simulink model "Main_C0_C3"  (R2023a)
(part 2 of 37)

  Left T Spine : sm_lib/Body Elements/File Solid  ExtGeomFileName=C:\Users\siril\OneDrive\Desktop\TIM-Control\Matlab\Simscape models\CAD - with COM\SymmetricModel\draft7\LeftThoracicSpineWithRibcage.step  UnitType=FromFile  ExtGeomFileUnits=m  StepReaderType=HEX  ExportConvexHullGeometry=off  InertiaType=CalculateFromGeometry  Mass=1  MassUnits=kg  CenterOfMass=[0 0 0]  CenterOfMassUnits=m  MomentsOfInertia=[1 1 1]  MomentsOfInertiaUnits=kg*m^2  ProductsOfInertia=[0 0 0]  ProductsOfInertiaUnits=kg*m^2  BasedOnType=Density  Density=0.182  DensityUnits=g/cm^3  DoExposeReferenceFrame=off  SerializedFrames=<Frames><Frame><Id>Frame1</Id><Value><Name>To L1</Name><Origin><Source>GeometricFeature</Source><FeatureName>segment 762</FeatureName></Origin><PrimaryAxis><DefinedDirection>-Z</DefinedDirection><Source>GeometricFeature</Source><SourceDirection>+Z</SourceDirection><FeatureName>planar surface 1266</FeatureName></PrimaryAxis><SecondaryAxis><DefinedDirection>+X</DefinedDirection><Source>ReferenceFrame</Source><SourceDirection>+X</SourceDirection><FeatureName></FeatureName></SecondaryAxis></Value></Frame><Frame><Id>Frame2</Id><Value><Name>To Left Abdominal Muscle</Name><Origin><Source>GeometricFeature</Source><FeatureName>planar surface 54556</FeatureName></Origin><PrimaryAxis><DefinedDirection>+Z</DefinedDirection><Source>GeometricFeature</Source><SourceDirection>+Z</SourceDirection><FeatureName>planar surface 54556</FeatureName></PrimaryAxis><SecondaryAxis><DefinedDirection>+X</DefinedDirection><Source>ReferenceFrame</Source><SourceDirection>+X</SourceDirection><FeatureName></FeatureName></SecondaryAxis></Value></Frame><Frame><Id>Frame3</Id><Value><Name>To Left Back Muscle</Name><Origin><Source>GeometricFeature</Source><FeatureName>planar surface 54574</FeatureName></Origin><PrimaryAxis><DefinedDirection>-Z</DefinedDirection><Source>GeometricFeature</Source><SourceDirection>+Z</SourceDirection><FeatureName>planar surface 54574</FeatureName></PrimaryAxis><SecondaryAxis><DefinedDirection>+X</DefinedDirection><Source>ReferenceFrame</Source><SourceDirection>+X</SourceDirection><FeatureName></FeatureName></SecondaryAxis></Value></Frame><Frame><Id>Frame4</Id><Value><Name>To Left Transverse1 Muscle</Name><Origin><Source>GeometricFeature</Source><FeatureName>planar surface 54586</FeatureName></Origin><PrimaryAxis><DefinedDirection>+Z</DefinedDirection><Source>GeometricFeature</Source><SourceDirection>+Z</SourceDirection><FeatureName>planar surface 54586</FeatureName></PrimaryAxis><SecondaryAxis><DefinedDirection>+X</DefinedDirection><Source>ReferenceFrame</Source><SourceDirection>+X</SourceDirection><FeatureName></FeatureName></SecondaryAxis></Value></Frame><Frame><Id>Frame5</Id><Value><Name>To Left Transverse2 Muscle</Name><Origin><Source>GeometricFeature</Source><FeatureName>planar surface 54611</FeatureName></Origin><PrimaryAxis><DefinedDirection>+Z</DefinedDirection><Source>GeometricFeature</Source><SourceDirection>+Z</SourceDirection><FeatureName>planar surface 54611</FeatureName></PrimaryAxis><SecondaryAxis><DefinedDirection>+X</DefinedDirection><Source>ReferenceFrame</Source><SourceDirection>+X</SourceDirection><FeatureName></FeatureName></SecondaryAxis></Value></Frame><Frame><Id>Frame6</Id><Value><Name>E01_Left_End_onTSpine</Name><Origin><Source>GeometricFeature</Source><FeatureName>point 64319</FeatureName></Origin><PrimaryAxis><DefinedDirection>+Z</DefinedDirection><Source>ReferenceFrame</Source><SourceDirection>+Z</SourceDirection><FeatureName></FeatureName></PrimaryAxis><SecondaryAxis><DefinedDirection>+X</DefinedDirection><Source>ReferenceFrame</Source><SourceDirection>+X</SourceDirection><FeatureName></FeatureName></SecondaryAxis></Value></Frame><Frame><Id>Frame7</Id><Value><Name>E02_Left_End_onTSpine</Name><Origin><Source>GeometricFeature</Source><FeatureName>point 57959</FeatureName></Origin><PrimaryAxis><DefinedDirection>+Z</DefinedDirection><Source>ReferenceFrame</Source><SourceDirection>+Z</SourceDirection><FeatureName></FeatureName></PrimaryAxis><SecondaryAxis><DefinedDirection>+X</DefinedDirection><Source>ReferenceFrame</Source><SourceDirection>+X</SourceDirection><FeatureName></FeatureName></SecondaryAxis></Value></Frame><Frame><Id>Frame8</Id><Value><Name>IO1_Left_End_onTSpine</Name><Origin><Source>GeometricFeature</Source><FeatureName>point 6575</FeatureName></Origin><PrimaryAxis><DefinedDirection>+Z</DefinedDirection><Source>ReferenceFrame</Source><SourceDirection>+Z</SourceDirection><FeatureName></FeatureName></PrimaryAxis><SecondaryAxis><DefinedDirection>+X</DefinedDirection><Source>ReferenceFrame</Source><SourceDirection>+X</SourceDirection><FeatureName></FeatureName></SecondaryAxis></Value></Frame><Frame><Id>Frame9</Id><Value><Name>IO2_Left_End_onTSpine</Name><Origin><Source>GeometricFeature</Source><FeatureName>point 61983</FeatureName></Origin><PrimaryAxis><DefinedDirection>+Z</DefinedDirection><Source>ReferenceFrame</Source><SourceDirection>+Z</SourceDirection><FeatureName></FeatureName></PrimaryAxis><SecondaryAxis><DefinedDirection>+X</DefinedDirection><Source>ReferenceFrame</Source><SourceDirection>+X</SourceDirection><FeatureName></FeatureName></SecondaryAxis></Value></Frame><Frame><Id>Frame10</Id><Value><Name>IO3_Left_End_onTSpine</Name><Origin><Source>GeometricFeature</Source><FeatureName>point 63240</FeatureName></Origin><PrimaryAxis><DefinedDirection>+Z</DefinedDirection><Source>ReferenceFrame</Source><SourceDirection>+Z</SourceDirection><FeatureName></FeatureName></PrimaryAxis><SecondaryAxis><DefinedDirection>+X</DefinedDirection><Source>ReferenceFrame</Source><SourceDirection>+X</SourceDirection><FeatureName></FeatureName></SecondaryAxis></Value></Frame><Frame><Id>Frame11</Id><Value><Name>To Left Clavicle</Name><Origin><Source>GeometricFeature</Source><FeatureName>point 134733</FeatureName></Origin><PrimaryAxis><DefinedDirection>+Z</DefinedDirection><Source>ReferenceFrame</Source><SourceDirection>+Z</SourceDirection><FeatureName></FeatureName></PrimaryAxis><SecondaryAxis><DefinedDirection>+X</DefinedDirection><Source>ReferenceFrame</Source><SourceDirection>+X</SourceDirection><FeatureName></FeatureName></SecondaryAxis></Value></Frame><Frame><Id>Frame12</Id><Value><Name>Left Lat1 Wrap1</Name><Origin><Source>GeometricFeature</Source><FeatureName>point 74792</FeatureName></Origin><PrimaryAxis><DefinedDirection>+Z</DefinedDirection><Source>ReferenceFrame</Source><SourceDirection>+Z</SourceDirection><FeatureName></FeatureName></PrimaryAxis><SecondaryAxis><DefinedDirection>+X</DefinedDirection><Source>ReferenceFrame</Source><SourceDirection>+X</SourceDirection><FeatureName></FeatureName></SecondaryAxis></Value></Frame><Frame><Id>Frame13</Id><Value><Name>Left Lat2 Wrap1</Name><Origin><Source>GeometricFeature</Source><FeatureName>point 104537</FeatureName></Origin><PrimaryAxis><DefinedDirection>+Z</DefinedDirection><Source>ReferenceFrame</Source><SourceDirection>+Z</SourceDirection><FeatureName></FeatureName></PrimaryAxis><SecondaryAxis><DefinedDirection>+X</DefinedDirection><Source>ReferenceFrame</Source><SourceDirection>+X</SourceDirection><FeatureName></FeatureName></SecondaryAxis></Value></Frame><Frame><Id>Frame14</Id><Value><Name>Left Lat1 Wrap2</Name><Origin><Source>GeometricFeature</Source><FeatureName>point 107483</FeatureName></Origin><PrimaryAxis><DefinedDirection>+Z</DefinedDirection><Source>ReferenceFrame</Source><SourceDirection>+Z</SourceDirection><FeatureName></FeatureName></PrimaryAxis><SecondaryAxis><DefinedDirection>+X</DefinedDirection><Source>ReferenceFrame</Source><SourceDirection>+X</SourceDirection><FeatureName></FeatureName></SecondaryAxis></Value></Frame><Frame><Id>Frame15</Id><Value><Name>Left Lat2 Wrap2</Name><Origin><Source>GeometricFeature</Source><FeatureName>point 35207</FeatureName></Origin><PrimaryAxis><DefinedDirection>+Z</DefinedDirection><Source>ReferenceFrame</Source><SourceDirection>+Z</SourceDirection><FeatureName></FeatureName></PrimaryAxis><SecondaryAxis><DefinedDirection>+X</DefinedDirection><Source>ReferenceFrame</Source><SourceDirection>+X</SourceDirection><FeatureName></FeatureName></SecondaryAxis></Value></Frame><Frame><Id>Frame16</Id><Value><Name>Left Lat3 Wrap1</Name><Origin><Source>GeometricFeature</Source><FeatureName>point 22410</FeatureName></Origin><PrimaryAxis><DefinedDirection>+Z</DefinedDirection><Source>ReferenceFrame</Source><SourceDirection>+Z</SourceDirection><FeatureName></FeatureName></PrimaryAxis><SecondaryAxis><DefinedDirection>+X</DefinedDirection><Source>ReferenceFrame</Source><SourceDirection>+X</SourceDirection><FeatureName></FeatureName></SecondaryAxis></Value></Frame></Frames>  GraphicType=FromGeometry  MarkerShape=Sphere  MarkerSize=10  GraphicVisPropType=SimpleVisualProperties  GraphicDiffuseColor=[0.84313726 0.8156863 0.7529412]  GraphicSpecularColor=[0.5 0.5 0.5 1.0]  GraphicAmbientColor=[0.15 0.15 0.15 1.0]  GraphicEmissiveColor=[0.0 0.0 0.0 1.0]  GraphicShininess=75  GraphicOpacity=1.0
  Left and Right Intertransverse Ligaments : Subsystem
  Mechanism Configuration : sm_lib/Utilities/Mechanism Configuration  UniformGravity=Constant  GravityVector=[0 0 -9.80665]  GravityVectorUnits=m/s^2  LinearizationDelta=0.001  JointModeTransitionNonlinearIterations=2
  Multiply21 : Gain  Gain=-1
  Muscle Forces : Subsystem
  PS-Simulink Converter{,1..6,8..39} (39 alike) : nesl_utility/PS-Simulink Converter  PhysicalDomain=network_engine_domain  SubClassName=ps_output  LeftPortType=input  RightPortType=output  PseudoPeriodic=off  Frequencies=[]  VectorFormat=inherit  Unit=inherit  AffineConversion=off
  Pure AR Moment at L1 COM : sm_lib/Forces and Torques/External Force and Torque  ForceResolutionFrame=World  EnableForceX=off  EnableForceY=off  EnableForceZ=off  EnableForce=off  TorqueResolutionFrame=World  EnableTorqueX=off  EnableTorqueY=off  EnableTorqueZ=on  EnableTorque=off
  Pure FE Moment at L1 COM : sm_lib/Forces and Torques/External Force and Torque  ForceResolutionFrame=World  EnableForceX=off  EnableForceY=off  EnableForceZ=off  EnableForce=off  TorqueResolutionFrame=World  EnableTorqueX=on  EnableTorqueY=off  EnableTorqueZ=off  EnableTorque=off
  Pure LB Moment at L1 COM : sm_lib/Forces and Torques/External Force and Torque  ForceResolutionFrame=World  EnableForceX=off  EnableForceY=off  EnableForceZ=off  EnableForce=off  TorqueResolutionFrame=World  EnableTorqueX=off  EnableTorqueY=on  EnableTorqueZ=off  EnableTorque=off
  Radians to Degrees3 : simulink_extras/Transformations/Radians to Degrees
  Radians to Degrees9 : simulink_extras/Transformations/Radians to Degrees
  Right T Spine : sm_lib/Body Elements/File Solid  ExtGeomFileName=C:\Users\siril\OneDrive\Desktop\TIM-Control\Matlab\Simscape models\CAD - with COM\SymmetricModel\draft7\RightThoracicSpineWithRibcage.step  UnitType=FromFile  ExtGeomFileUnits=m  StepReaderType=HEX  ExportConvexHullGeometry=off  InertiaType=CalculateFromGeometry  Mass=1  MassUnits=kg  CenterOfMass=[0 0 0]  CenterOfMassUnits=m  MomentsOfInertia=[1 1 1]  MomentsOfInertiaUnits=kg*m^2  ProductsOfInertia=[0 0 0]  ProductsOfInertiaUnits=kg*m^2  BasedOnType=Density  Density=0.182  DensityUnits=g/cm^3  DoExposeReferenceFrame=off  SerializedFrames=<Frames><Frame><Id>Frame1</Id><Value><Name>To L1</Name><Origin><Source>GeometricFeature</Source><FeatureName>segment 633</FeatureName></Origin><PrimaryAxis><DefinedDirection>+Z</DefinedDirection><Source>GeometricFeature</Source><SourceDirection>+Z</SourceDirection><FeatureName>planar surface 1266</FeatureName></PrimaryAxis><SecondaryAxis><DefinedDirection>+X</DefinedDirection><Source>ReferenceFrame</Source><SourceDirection>+X</SourceDirection><FeatureName></FeatureName></SecondaryAxis></Value></Frame><Frame><Id>Frame2</Id><Value><Name>To Right Abdominal Muscle</Name><Origin><Source>GeometricFeature</Source><FeatureName>planar surface 54556</FeatureName></Origin><PrimaryAxis><DefinedDirection>-Z</DefinedDirection><Source>GeometricFeature</Source><SourceDirection>+Z</SourceDirection><FeatureName>planar surface 54556</FeatureName></PrimaryAxis><SecondaryAxis><DefinedDirection>+X</DefinedDirection><Source>ReferenceFrame</Source><SourceDirection>+X</SourceDirection><FeatureName></FeatureName></SecondaryAxis></Value></Frame><Frame><Id>Frame3</Id><Value><Name>To Right Back Muscle</Name><Origin><Source>GeometricFeature</Source><FeatureName>planar surface 54574</FeatureName></Origin><PrimaryAxis><DefinedDirection>+Z</DefinedDirection><Source>GeometricFeature</Source><SourceDirection>+Z</SourceDirection><FeatureName>planar surface 54574</FeatureName></PrimaryAxis><SecondaryAxis><DefinedDirection>+X</DefinedDirection><Source>ReferenceFrame</Source><SourceDirection>+X</SourceDirection><FeatureName></FeatureName></SecondaryAxis></Value></Frame><Frame><Id>Frame4</Id><Value><Name>To Right Transverse1 Muscle</Name><Origin><Source>GeometricFeature</Source><FeatureName>planar surface 54586</FeatureName></Origin><PrimaryAxis><DefinedDirection>-Z</DefinedDirection><Source>GeometricFeature</Source><SourceDirection>+Z</SourceDirection><FeatureName>planar surface 54586</FeatureName></PrimaryAxis><SecondaryAxis><DefinedDirection>+X</DefinedDirection><Source>ReferenceFrame</Source><SourceDirection>+X</SourceDirection><FeatureName></FeatureName></SecondaryAxis></Value></Frame><Frame><Id>Frame5</Id><Value><Name>To Right Transverse2 Muscle</Name><Origin><Source>GeometricFeature</Source><FeatureName>planar surface 54611</FeatureName></Origin><PrimaryAxis><DefinedDirection>-Z</DefinedDirection><Source>GeometricFeature</Source><SourceDirection>+Z</SourceDirection><FeatureName>planar surface 54611</FeatureName></PrimaryAxis><SecondaryAxis><DefinedDirection>+X</DefinedDirection><Source>ReferenceFrame</Source><SourceDirection>+X</SourceDirection><FeatureName></FeatureName></SecondaryAxis></Value></Frame><Frame><Id>Frame6</Id><Value><Name>T1 Plumbline Frame</Name><Origin><Source>GeometricFeature</Source><FeatureName>point 5793</FeatureName></Origin><PrimaryAxis><DefinedDirection>+Z</DefinedDirection><Source>ReferenceFrame</Source><SourceDirection>+Z</SourceDirection><FeatureName></FeatureName></PrimaryAxis><SecondaryAxis><DefinedDirection>+X</DefinedDirection><Source>ReferenceFrame</Source><SourceDirection>+X</SourceDirection><FeatureName></FeatureName></SecondaryAxis></Value></Frame><Frame><Id>Frame7</Id><Value><Name>T5 Spinous Process Tip</Name><Origin><Source>GeometricFeature</Source><FeatureName>point 6426</FeatureName></Origin><PrimaryAxis><DefinedDirection>+Z</DefinedDirection><Source>ReferenceFrame</Source><SourceDirection>+Z</SourceDirection><FeatureName></FeatureName></PrimaryAxis><SecondaryAxis><DefinedDirection>+X</DefinedDirection><Source>ReferenceFrame</Source><SourceDirection>+X</SourceDirection><FeatureName></FeatureName></SecondaryAxis></Value></Frame><Frame><Id>Frame8</Id><Value><Name>T1 Spinous Process Tip</Name><Origin><Source>GeometricFeature</Source><FeatureName>point 327</FeatureName></Origin><PrimaryAxis><DefinedDirection>+Z</DefinedDirection><Source>ReferenceFrame</Source><SourceDirection>+Z</SourceDirection><FeatureName></FeatureName></PrimaryAxis><SecondaryAxis><DefinedDirection>+X</DefinedDirection><Source>ReferenceFrame</Source><SourceDirection>+X</SourceDirection><FeatureName></FeatureName></SecondaryAxis></Value></Frame><Frame><Id>Frame9</Id><Value><Name>T10 Spinous process tip</Name><Origin><Source>GeometricFeature</Source><FeatureName>point 46212</FeatureName></Origin><PrimaryAxis><DefinedDirection>+Z</DefinedDirection><Source>ReferenceFrame</Source><SourceDirection>+Z</SourceDirection><FeatureName></FeatureName></PrimaryAxis><SecondaryAxis><DefinedDirection>+X</DefinedDirection><Source>ReferenceFrame</Source><SourceDirection>+X</SourceDirection><FeatureName></FeatureName></SecondaryAxis></Value></Frame><Frame><Id>Frame10</Id><Value><Name>T12 Spinous Process tip</Name><Origin><Source>GeometricFeature</Source><FeatureName>point 4338</FeatureName></Origin><PrimaryAxis><DefinedDirection>+Z</DefinedDirection><Source>ReferenceFrame</Source><SourceDirection>+Z</SourceDirection><FeatureName></FeatureName></PrimaryAxis><SecondaryAxis><DefinedDirection>+X</DefinedDirection><Source>ReferenceFrame</Source><SourceDirection>+X</SourceDirection><FeatureName></FeatureName></SecondaryAxis></Value></Frame><Frame><Id>Frame11</Id><Value><Name>E01_Right_End_onTSpine</Name><Origin><Source>GeometricFeature</Source><FeatureName>point 58766</FeatureName></Origin><PrimaryAxis><DefinedDirection>+Z</DefinedDirection><Source>ReferenceFrame</Source><SourceDirection>+Z</SourceDirection><FeatureName></FeatureName></PrimaryAxis><SecondaryAxis><DefinedDirection>+X</DefinedDirection><Source>ReferenceFrame</Source><SourceDirection>+X</SourceDirection><FeatureName></FeatureName></SecondaryAxis></Value></Frame><Frame><Id>Frame12</Id><Value><Name>E02_Right_End_onTSpine</Name><Origin><Source>GeometricFeature</Source><FeatureName>point 57959</FeatureName></Origin><PrimaryAxis><DefinedDirection>+Z</DefinedDirection><Source>ReferenceFrame</Source><SourceDirection>+Z</SourceDirection><FeatureName></FeatureName></PrimaryAxis><SecondaryAxis><DefinedDirection>+X</DefinedDirection><Source>ReferenceFrame</Source><SourceDirection>+X</SourceDirection><FeatureName></FeatureName></SecondaryAxis></Value></Frame><Frame><Id>Frame13</Id><Value><Name>IO1_Right_End_onTSpine</Name><Origin><Source>GeometricFeature</Source><FeatureName>point 6577</FeatureName></Origin><PrimaryAxis><DefinedDirection>+Z</DefinedDirection><Source>ReferenceFrame</Source><SourceDirection>+Z</SourceDirection><FeatureName></FeatureName></PrimaryAxis><SecondaryAxis><DefinedDirection>+X</DefinedDirection><Source>ReferenceFrame</Source><SourceDirection>+X</SourceDirection><FeatureName></FeatureName></SecondaryAxis></Value></Frame><Frame><Id>Frame14</Id><Value><Name>IO2_Right_End_onTSpine</Name><Origin><Source>GeometricFeature</Source><FeatureName>point 61985</FeatureName></Origin><PrimaryAxis><DefinedDirection>+Z</DefinedDirection><Source>ReferenceFrame</Source><SourceDirection>+Z</SourceDirection><FeatureName></FeatureName></PrimaryAxis><SecondaryAxis><DefinedDirection>+X</DefinedDirection><Source>ReferenceFrame</Source><SourceDirection>+X</SourceDirection><FeatureName></FeatureName></SecondaryAxis></Value></Frame><Frame><Id>Frame15</Id><Value><Name>IO3_Right_End_onTSpine</Name><Origin><Source>GeometricFeature</Source><FeatureName>point 63240</FeatureName></Origin><PrimaryAxis><DefinedDirection>+Z</DefinedDirection><Source>ReferenceFrame</Source><SourceDirection>+Z</SourceDirection><FeatureName></FeatureName></PrimaryAxis><SecondaryAxis><DefinedDirection>+X</DefinedDirection><Source>ReferenceFrame</Source><SourceDirection>+X</SourceDirection><FeatureName></FeatureName></SecondaryAxis></Value></Frame><Frame><Id>Frame16</Id><Value><Name>To Clavicle</Name><Origin><Source>GeometricFeature</Source><FeatureName>point 134734</FeatureName></Origin><PrimaryAxis><DefinedDirection>+Z</DefinedDirection><Source>ReferenceFrame</Source><SourceDirection>+Z</SourceDirection><FeatureName></FeatureName></PrimaryAxis><SecondaryAxis><DefinedDirection>+X</DefinedDirection><Source>ReferenceFrame</Source><SourceDirection>+X</SourceDirection><FeatureName></FeatureName></SecondaryAxis></Value></Frame><Frame><Id>Frame18</Id><Value><Name>Right Lat2 Wrap1</Name><Origin><Source>GeometricFeature</Source><FeatureName>point 104540</FeatureName></Origin><PrimaryAxis><DefinedDirection>+Z</DefinedDirection><Source>ReferenceFrame</Source><SourceDirection>+Z</SourceDirection><FeatureName></FeatureName></PrimaryAxis><SecondaryAxis><DefinedDirection>+X</DefinedDirection><Source>ReferenceFrame</Source><SourceDirection>+X</SourceDirection><FeatureName></FeatureName></SecondaryAxis></Value></Frame><Frame><Id>Frame19</Id><Value><Name>Right Lat3 Wrap1</Name><Origin><Source>GeometricFeature</Source><FeatureName>point 112273</FeatureName></Origin><PrimaryAxis><DefinedDirection>+Z</DefinedDirection><Source>ReferenceFrame</Source><SourceDirection>+Z</SourceDirection><FeatureName></FeatureName></PrimaryAxis><SecondaryAxis><DefinedDirection>+X</DefinedDirection><Source>ReferenceFrame</Source><SourceDirection>+X</SourceDirection><FeatureName></FeatureName></SecondaryAxis></Value></Frame><Frame><Id>Frame20</Id><Value><Name>Right Lat1 Wrap1</Name><Origin><Source>GeometricFeature</Source><FeatureName>point 74799</FeatureName></Origin><PrimaryAxis><DefinedDirection>+Z</DefinedDirection><Source>ReferenceFrame</Source><SourceDirection>+Z</SourceDirection><FeatureName></FeatureName></PrimaryAxis><SecondaryAxis><DefinedDirection>+X</DefinedDirection><Source>ReferenceFrame</Source><SourceDirection>+X</SourceDirection><FeatureName></FeatureName></SecondaryAxis></Value></Frame><Frame><Id>Frame21</Id><Value><Name>Right Lat2 Wrap2</Name><Origin><Source>GeometricFeature</Source><FeatureName>point 35221</FeatureName></Origin><PrimaryAxis><DefinedDirection>+Z</DefinedDirection><Source>ReferenceFrame</Source><SourceDirection>+Z</SourceDirection><FeatureName></FeatureName></PrimaryAxis><SecondaryAxis><DefinedDirection>+X</DefinedDirection><Source>ReferenceFrame</Source><SourceDirection>+X</SourceDirection><FeatureName></FeatureName></SecondaryAxis></Value></Frame><Frame><Id>Frame22</Id><Value><Name>Right Lat1 Wrap2</Name><Origin><Source>GeometricFeature</Source><FeatureName>point 107483</FeatureName></Origin><PrimaryAxis><DefinedDirection>+Z</DefinedDirection><Source>ReferenceFrame</Source><SourceDirection>+Z</SourceDirection><FeatureName></FeatureName></PrimaryAxis><SecondaryAxis><DefinedDirection>+X</DefinedDirection><Source>ReferenceFrame</Source><SourceDirection>+X</SourceDirection><FeatureName></FeatureName></SecondaryAxis></Value></Frame></Frames>  GraphicType=FromGeometry  MarkerShape=Sphere  MarkerSize=10  GraphicVisPropType=SimpleVisualProperties  GraphicDiffuseColor=[0.84313726 0.8156863 0.7529412]  GraphicSpecularColor=[0.5 0.5 0.5 1.0]  GraphicAmbientColor=[0.15 0.15 0.15 1.0]  GraphicEmissiveColor=[0.0 0.0 0.0 1.0]  GraphicShininess=75  GraphicOpacity=1.0
  S1 : sm_lib/Body Elements/File Solid  ExtGeomFileName=C:\Users\siril\OneDrive\Desktop\TIM-Control\Matlab\Simscape models\Reduced Order Model\CAD\model without nucleus\S1.step  UnitType=FromFile  ExtGeomFileUnits=m  StepReaderType=HEX  ExportConvexHullGeometry=off  InertiaType=CalculateFromGeometry  Mass=1  MassUnits=kg  CenterOfMass=[0 0 0]  CenterOfMassUnits=m  MomentsOfInertia=[1 1 1]  MomentsOfInertiaUnits=kg*m^2  ProductsOfInertia=[0 0 0]  ProductsOfInertiaUnits=kg*m^2  BasedOnType=Density  Density=0.182  DensityUnits=g/cm^3  DoExposeReferenceFrame=on  SerializedFrames=<Frames><Frame><Id>Frame1</Id><Value><Name>to IVD5</Name><Origin><Source>GeometricFeature</Source><FeatureName>planar surface 12322</FeatureName></Origin><PrimaryAxis><DefinedDirection>+Z</DefinedDirection><Source>GeometricFeature</Source><SourceDirection>+Z</SourceDirection><FeatureName>planar surface 12322</FeatureName></PrimaryAxis><SecondaryAxis><DefinedDirection>+X</DefinedDirection><Source>ReferenceFrame</Source><SourceDirection>+X</SourceDirection><FeatureName></FeatureName></SecondaryAxis></Value></Frame><Frame><Id>Frame2</Id><Value><Name>For Plumbline Evaluation</Name><Origin><Source>GeometricFeature</Source><FeatureName>planar surface 2453</FeatureName></Origin><PrimaryAxis><DefinedDirection>+Y</DefinedDirection><Source>GeometricFeature</Source><SourceDirection>+Z</SourceDirection><FeatureName>planar surface 2453</FeatureName></PrimaryAxis><SecondaryAxis><DefinedDirection>+X</DefinedDirection><Source>ReferenceFrame</Source><SourceDirection>+X</SourceDirection><FeatureName></FeatureName></SecondaryAxis></Value></Frame><Frame><Id>Frame3</Id><Value><Name>To Right Abdominal Muscle</Name><Origin><Source>GeometricFeature</Source><FeatureName>planar surface 11971</FeatureName></Origin><PrimaryAxis><DefinedDirection>-Z</DefinedDirection><Source>GeometricFeature</Source><SourceDirection>+Z</SourceDirection><FeatureName>planar surface 11971</FeatureName></PrimaryAxis><SecondaryAxis><DefinedDirection>+X</DefinedDirection><Source>ReferenceFrame</Source><SourceDirection>+X</SourceDirection><FeatureName></FeatureName></SecondaryAxis></Value></Frame><Frame><Id>Frame4</Id><Value><Name>To Right Transverse2 Muscle</Name><Origin><Source>GeometricFeature</Source><FeatureName>planar surface 39</FeatureName></Origin><PrimaryAxis><DefinedDirection>-Z</DefinedDirection><Source>GeometricFeature</Source><SourceDirection>+Z</SourceDirection><FeatureName>planar surface 39</FeatureName></PrimaryAxis><SecondaryAxis><DefinedDirection>+X</DefinedDirection><Source>ReferenceFrame</Source><SourceDirection>+X</SourceDirection><FeatureName></FeatureName></SecondaryAxis></Value></Frame><Frame><Id>Frame5</Id><Value><Name>To Right Transverse1 Muscle</Name><Origin><Source>GeometricFeature</Source><FeatureName>planar surface 53</FeatureName></Origin><PrimaryAxis><DefinedDirection>-Z</DefinedDirection><Source>GeometricFeature</Source><SourceDirection>+Z</SourceDirection><FeatureName>planar surface 53</FeatureName></PrimaryAxis><SecondaryAxis><DefinedDirection>+X</DefinedDirection><Source>ReferenceFrame</Source><SourceDirection>+X</SourceDirection><FeatureName></FeatureName></SecondaryAxis></Value></Frame><Frame><Id>Frame6</Id><Value><Name>To Right Back Muscle</Name><Origin><Source>GeometricFeature</Source><FeatureName>planar surface 11999</FeatureName></Origin><PrimaryAxis><DefinedDirection>-Z</DefinedDirection><Source>GeometricFeature</Source><SourceDirection>+Z</SourceDirection><FeatureName>planar surface 11999</FeatureName></PrimaryAxis><SecondaryAxis><DefinedDirection>+X</DefinedDirection><Source>ReferenceFrame</Source><SourceDirection>+X</SourceDirection><FeatureName></FeatureName></SecondaryAxis></Value></Frame><Frame><Id>Frame7</Id><Value><Name>To Left Back Muscle</Name><Origin><Source>GeometricFeature</Source><FeatureName>planar surface 7087</FeatureName></Origin><PrimaryAxis><DefinedDirection>+Z</DefinedDirection><Source>GeometricFeature</Source><SourceDirection>+Z</SourceDirection><FeatureName>planar surface 7087</FeatureName></PrimaryAxis><SecondaryAxis><DefinedDirection>+X</DefinedDirection><Source>ReferenceFrame</Source><SourceDirection>+X</SourceDirection><FeatureName></FeatureName></SecondaryAxis></Value></Frame><Frame><Id>Frame8</Id><Value><Name>To Left Transverse1 Muscle</Name><Origin><Source>GeometricFeature</Source><FeatureName>planar surface 2357</FeatureName></Origin><PrimaryAxis><DefinedDirection>+Z</DefinedDirection><Source>GeometricFeature</Source><SourceDirection>+Z</SourceDirection><FeatureName>planar surface 2357</FeatureName></PrimaryAxis><SecondaryAxis><DefinedDirection>+X</DefinedDirection><Source>ReferenceFrame</Source><SourceDirection>+X</SourceDirection><FeatureName></FeatureName></SecondaryAxis></Value></Frame><Frame><Id>Frame9</Id><Value><Name>To Left Transverse2 Muscle</Name><Origin><Source>GeometricFeature</Source><FeatureName>planar surface 2371</FeatureName></Origin><PrimaryAxis><DefinedDirection>+Z</DefinedDirection><Source>GeometricFeature</Source><SourceDirection>+Z</SourceDirection><FeatureName>planar surface 2371</FeatureName></PrimaryAxis><SecondaryAxis><DefinedDirection>+X</DefinedDirection><Source>ReferenceFrame</Source><SourceDirection>+X</SourceDirection><FeatureName></FeatureName></SecondaryAxis></Value></Frame><Frame><Id>Frame10</Id><Value><Name>To Left Abdominal Muscle</Name><Origin><Source>GeometricFeature</Source><FeatureName>planar surface 7059</FeatureName></Origin><PrimaryAxis><DefinedDirection>+Z</DefinedDirection><Source>GeometricFeature</Source><SourceDirection>+Z</SourceDirection><FeatureName>planar surface 7059</FeatureName></PrimaryAxis><SecondaryAxis><DefinedDirection>+X</DefinedDirection><Source>ReferenceFrame</Source><SourceDirection>+X</SourceDirection><FeatureName></FeatureName></SecondaryAxis></Value></Frame><Frame><Id>Frame11</Id><Value><Name>To L5 SSL</Name><Origin><Source>GeometricFeature</Source><FeatureName>point 40698</FeatureName></Origin><PrimaryAxis><DefinedDirection>+Z</DefinedDirection><Source>ReferenceFrame</Source><SourceDirection>+Z</SourceDirection><FeatureName></FeatureName></PrimaryAxis><SecondaryAxis><DefinedDirection>+X</DefinedDirection><Source>ReferenceFrame</Source><SourceDirection>+X</SourceDirection><FeatureName></FeatureName></SecondaryAxis></Value></Frame><Frame><Id>Frame12</Id><Value><Name>To L5 ISL</Name><Origin><Source>GeometricFeature</Source><FeatureName>point 40776</FeatureName></Origin><PrimaryAxis><DefinedDirection>+Z</DefinedDirection><Source>ReferenceFrame</Source><SourceDirection>+Z</SourceDirection><FeatureName></FeatureName></PrimaryAxis><SecondaryAxis><DefinedDirection>+X</DefinedDirection><Source>ReferenceFrame</Source><SourceDirection>+X</SourceDirection><FeatureName></FeatureName></SecondaryAxis></Value></Frame><Frame><Id>Frame13</Id><Value><Name>To Right L5 ITL</Name><Origin><Source>GeometricFeature</Source><FeatureName>point 2768</FeatureName></Origin><PrimaryAxis><DefinedDirection>+Z</DefinedDirection><Source>ReferenceFrame</Source><SourceDirection>+Z</SourceDirection><FeatureName></FeatureName></PrimaryAxis><SecondaryAxis><DefinedDirection>+X</DefinedDirection><Source>ReferenceFrame</Source><SourceDirection>+X</SourceDirection><FeatureName></FeatureName></SecondaryAxis></Value></Frame><Frame><Id>Frame14</Id><Value><Name>To Left L5 ITL</Name><Origin><Source>GeometricFeature</Source><FeatureName>point 5454</FeatureName></Origin><PrimaryAxis><DefinedDirection>+Z</DefinedDirection><Source>ReferenceFrame</Source><SourceDirection>+Z</SourceDirection><FeatureName></FeatureName></PrimaryAxis><SecondaryAxis><DefinedDirection>+X</DefinedDirection><Source>ReferenceFrame</Source><SourceDirection>+X</SourceDirection><FeatureName></FeatureName></SecondaryAxis></Value></Frame><Frame><Id>Frame15</Id><Value><Name>EO1_Left_Start_onS1</Name><Origin><Source>GeometricFeature</Source><FeatureName>point 6853</FeatureName></Origin><PrimaryAxis><DefinedDirection>+Z</DefinedDirection><Source>ReferenceFrame</Source><SourceDirection>+Z</SourceDirection><FeatureName></FeatureName></PrimaryAxis><SecondaryAxis><DefinedDirection>+X</DefinedDirection><Source>ReferenceFrame</Source><SourceDirection>+X</SourceDirection><FeatureName></FeatureName></SecondaryAxis></Value></Frame><Frame><Id>Frame16</Id><Value><Name>EO2_Left_Start_onS1</Name><Origin><Source>GeometricFeature</Source><FeatureName>point 6794</FeatureName></Origin><PrimaryAxis><DefinedDirection>+Z</DefinedDirection><Source>ReferenceFrame</Source><SourceDirection>+Z</SourceDirection><FeatureName></FeatureName></PrimaryAxis><SecondaryAxis><DefinedDirection>+X</DefinedDirection><Source>ReferenceFrame</Source><SourceDirection>+X</SourceDirection><FeatureName></FeatureName></SecondaryAxis></Value></Frame><Frame><Id>Frame17</Id><Value><Name>EO1_Right_Start_onS1</Name><Origin><Source>GeometricFeature</Source><FeatureName>point 1489</FeatureName></Origin><PrimaryAxis><DefinedDirection>+Z</DefinedDirection><Source>ReferenceFrame</Source><SourceDirection>+Z</SourceDirection><FeatureName></FeatureName></PrimaryAxis><SecondaryAxis><DefinedDirection>+X</DefinedDirection><Source>ReferenceFrame</Source><SourceDirection>+X</SourceDirection><FeatureName></FeatureName></SecondaryAxis></Value></Frame><Frame><Id>Frame18</Id><Value><Name>EO2_Right_Start_onS1</Name><Origin><Source>GeometricFeature</Source><FeatureName>point 1411</FeatureName></Origin><PrimaryAxis><DefinedDirection>+Z</DefinedDirection><Source>ReferenceFrame</Source><SourceDirection>+Z</SourceDirection><FeatureName></FeatureName></PrimaryAxis><SecondaryAxis><DefinedDirection>+X</DefinedDirection><Source>ReferenceFrame</Source><SourceDirection>+X</SourceDirection><FeatureName></FeatureName></SecondaryAxis></Value></Frame><Frame><Id>Frame19</Id><Value><Name>IO1_Right_Start_onS1</Name><Origin><Source>GeometricFeature</Source><FeatureName>point 1008</FeatureName></Origin><PrimaryAxis><DefinedDirection>+Z</DefinedDirection><Source>ReferenceFrame</Source><SourceDirection>+Z</SourceDirection><FeatureName></FeatureName></PrimaryAxis><SecondaryAxis><DefinedDirection>+X</DefinedDirection><Source>ReferenceFrame</Source><SourceDirection>+X</SourceDirection><FeatureName></FeatureName></SecondaryAxis></Value></Frame><Frame><Id>Frame20</Id><Value><Name>IO2_Right_Start_onS1</Name><Origin><Source>GeometricFeature</Source><FeatureName>point 1849</FeatureName></Origin><PrimaryAxis><DefinedDirection>+Z</DefinedDirection><Source>ReferenceFrame</Source><SourceDirection>+Z</SourceDirection><FeatureName></FeatureName></PrimaryAxis><SecondaryAxis><DefinedDirection>+X</DefinedDirection><Source>ReferenceFrame</Source><SourceDirection>+X</SourceDirection><FeatureName></FeatureName></SecondaryAxis></Value></Frame><Frame><Id>Frame21</Id><Value><Name>IO3_Right_Start_onS1</Name><Origin><Source>GeometricFeature</Source><FeatureName>point 1461</FeatureName></Origin><PrimaryAxis><DefinedDirection>+Z</DefinedDirection><Source>ReferenceFrame</Source><SourceDirection>+Z</SourceDirection><FeatureName></FeatureName></PrimaryAxis><SecondaryAxis><DefinedDirection>+X</DefinedDirection><Source>ReferenceFrame</Source><SourceDirection>+X</SourceDirection><FeatureName></FeatureName></SecondaryAxis></Value></Frame><Frame><Id>Frame22</Id><Value><Name>IO1_Left_Start_onS1</Name><Origin><Source>GeometricFeature</Source><FeatureName>point 6435</FeatureName></Origin><PrimaryAxis><DefinedDirection>+Z</DefinedDirection><Source>ReferenceFrame</Source><SourceDirection>+Z</SourceDirection><FeatureName></FeatureName></PrimaryAxis><SecondaryAxis><DefinedDirection>+X</DefinedDirection><Source>ReferenceFrame</Source><SourceDirection>+X</SourceDirection><FeatureName></FeatureName></SecondaryAxis></Value></Frame><Frame><Id>Frame23</Id><Value><Name>IO2_Left_Start_onS1</Name><Origin><Source>GeometricFeature</Source><FeatureName>point 6377</FeatureName></Origin><PrimaryAxis><DefinedDirection>+Z</DefinedDirection><Source>ReferenceFrame</Source><SourceDirection>+Z</SourceDirection><FeatureName></FeatureName></PrimaryAxis><SecondaryAxis><DefinedDirection>+X</DefinedDirection><Source>ReferenceFrame</Source><SourceDirection>+X</SourceDirection><FeatureName></FeatureName></SecondaryAxis></Value></Frame><Frame><Id>Frame24</Id><Value><Name>IO3_Left_Start_onS1</Name><Origin><Source>GeometricFeature</Source><FeatureName>point 6825</FeatureName></Origin><PrimaryAxis><DefinedDirection>+Z</DefinedDirection><Source>ReferenceFrame</Source><SourceDirection>+Z</SourceDirection><FeatureName></FeatureName></PrimaryAxis><SecondaryAxis><DefinedDirection>+X</DefinedDirection><Source>ReferenceFrame</Source><SourceDirection>+X</SourceDirection><FeatureName></FeatureName></SecondaryAxis></Value></Frame></Frames>  GraphicType=FromGeometry  MarkerShape=Sphere  MarkerSize=10  GraphicVisPropType=SimpleVisualProperties  GraphicDiffuseColor=[0.84313726 0.8156863 0.7529412]  GraphicSpecularColor=[0.5 0.5 0.5 1.0]  GraphicAmbientColor=[0.15 0.15 0.15 1.0]  GraphicEmissiveColor=[0.0 0.0 0.0 1.0]  GraphicShininess=75  GraphicOpacity=1.0
  Scope17 : Scope  NumInputPorts=5
  Scope{5..6,19..20} (4 alike) : Scope
  Simulink-PS Converter : nesl_utility/Simulink-PS Converter  Commented=on  PhysicalDomain=network_engine_domain  SubClassName=ps_input  LeftPortType=input  RightPortType=output  PseudoPeriodic=off  Frequencies=[]  NoiseDistribution=none  NoiseParameters=[]  Unit=1  AffineConversion=off  FilteringAndDerivatives=provide  SimscapeFilterOrder=1  InputFilterTimeConstant=0.001  UdotUserProvided=0
  Simulink-PS Converter{1..7} (7 alike) : nesl_utility/Simulink-PS Converter  PhysicalDomain=network_engine_domain  SubClassName=ps_input  LeftPortType=input  RightPortType=output  PseudoPeriodic=off  Frequencies=[]  NoiseDistribution=none  NoiseParameters=[]  Unit=1  AffineConversion=off  FilteringAndDerivatives=provide  SimscapeFilterOrder=1  InputFilterTimeConstant=0.001  UdotUserProvided=0
  Solver Configuration : nesl_utility/Solver Configuration  PhysicalDomain=network_engine_domain  SubClassName=solver  LeftPortType=input  RightPortType=generic  Tones=[]  Harmonics=[]  SimulateNoise=off  Profile=off  UseLocalSampling=off  EnableSwitchedLinearOptims=on  FrequencyDomain=off  UseCCode=off  RelTol=0.001  AbsTol=1e-06  MinStep=1e-09  ToWorkspace=off  RevertToSquareIcSolve=off  NumHomotopyIterations=100  PhasorMode=off  PhasorModeNumHarmonics=1  ConsistencySolver=NEWTON_FTOL  IndexReductionMethod=DerivativeReplacement  DoDC=off  ResidualTolerance=1e-02  ConsistencyTolSource=GLOBAL  ConsistencyAbsTol=0.001  ConsistencyRelTol=0.001  ConsistencyTolFactor=0.001  UseLocalSolver=off  LocalSolverChoice=NE_BACKWARD_EULER_ADVANCER  ResolveIndetEquations=on  FunctionEvalNumThread=1  LocalSolverSampleTime=0.001  DoFixedCost=off  MaxNonlinIter=3  MaxModeIter=2  ComputeImpulses=off  ImpulseIterations=2  LinearAlgebra=Sparse  LinearAlgebraNumThread=0  EquationFormulation=NE_TIME_EF  DelaysMemoryBudget=1024  AutomaticFiltering=on  FilteringTimeConstant=0.001  PartitionStorageMethod=AS_NEEDED  PartitionMemoryBudget=1024  PartitionMethod=FAST
  Subtract{,1..4} (5 alike) : Sum  Inputs=+-
  Supraspinous Ligaments : Subsystem
      settings: PortSchema="{\"entries\":[{\"content\":{\"sides\":[{\"content\":{\"connectorIds\":[\"LConn1\",\"LConn2\",\"LConn3\",\"LConn4\",\"LConn5\",\"LConn6\",\"LConn7\",\"LConn8\",\"LConn9\",\"LConn10\"]},\"type\":\"ConnectorPlacement.EquallySpacedRectSide\",\"uuid\":\"e07d9df3-a27b-4d09-b924-4f5a3ab18cb1\"},{\"content\":{\"side\":\"RIGHT\"},\"type\":\"ConnectorPlacement.EquallySpacedRectSide\",\"uuid\":\"03fb9f89-c758-4913-97e7-2cef46f04585\"},{\"content\":{\"side\":\"TOP\"},\"type\":\"ConnectorPlacement.EquallySpacedRectSide\",\"uuid\":\"345d4093-6760-4c36-a866-bd524106f5ee\"},{\"content\":{\"connectorIds\":[\"RConn1\"],\"side\":\"BOTTOM\"},\"type\":\"ConnectorPlacement.EquallySpacedRectSide\",\"uuid\":\"2235079a-702b-4d8f-85b3-5494ca7f0e19\"}]},\"type\":\"ConnectorPlacement.EquallySpacedConnector\",\"uuid\":\"01bb975a-4a91-480e-96d4-2d77fbdfd389\"}],\"packageUris\":[\"http://schema.mathworks.com/mf0/Connector/R2020b\"],\"version\":\"1.0\"}"
  T1-S1 Bushing Joint : sm_lib/Joints/Bushing Joint  JointMode=Normal  SenseConstraintForce=off  SenseConstraintForceX=off  SenseConstraintForceY=off  SenseConstraintForceZ=off  SenseConstraintTorque=off  SenseConstraintTorqueX=off  SenseConstraintTorqueY=off  SenseConstraintTorqueZ=off  SenseTotalForce=off  SenseTotalForceX=off  SenseTotalForceY=off  SenseTotalForceZ=off  SenseTotalTorque=off  SenseTotalTorqueX=off  SenseTotalTorqueY=off  SenseTotalTorqueZ=off  CompositeWrenchDir=FollowerOnBase  CompositeWrenchFrame=BaseFrame  PxEquilibriumPosition=0  PxEquilibriumPositionUnits=m  PxSpringStiffness=0  PxSpringStiffnessUnits=N/m  PxDampingCoefficient=0  PxDampingCoefficientUnits=N/(m/s)  PxTorqueActuationMode=NoTorque  PxMotionActuationMode=ComputedMotion  PxSensePosition=on  PxSenseVelocity=off  PxSenseAcceleration=off  PxSenseTorqueForce=off  PxSenseLowerLimitTorqueForce=off  PxSenseUpperLimitTorqueForce=off  PxLowerLimitSpecify=off  PxLowerLimitBound=-1  PxLowerLimitBoundUnits=m  PxLowerLimitStiffness=1e6  PxLowerLimitStiffnessUnits=N/m  PxLowerLimitDamping=1e3  PxLowerLimitDampingUnits=N/(m/s)  PxLowerLimitTransitionRegionWidth=1e-4  PxLowerLimitTransitionRegionWidthUnits=m  PxUpperLimitSpecify=off  PxUpperLimitBound=1  PxUpperLimitBoundUnits=m  PxUpperLimitStiffness=1e6  PxUpperLimitStiffnessUnits=N/m  PxUpperLimitDamping=1e3  PxUpperLimitDampingUnits=N/(m/s)  PxUpperLimitTransitionRegionWidth=1e-4  PxUpperLimitTransitionRegionWidthUnits=m  PxPositionTargetSpecify=off  PxPositionTargetPriority=High  PxPositionTargetValue=0  PxPositionTargetValueUnits=m  PxVelocityTargetSpecify=off  PxVelocityTargetPriority=High  PxVelocityTargetValue=0  PxVelocityTargetValueUnits=m/s  PyEquilibriumPosition=0  PyEquilibriumPositionUnits=m  PySpringStiffness=0  PySpringStiffnessUnits=N/m  PyDampingCoefficient=0  PyDampingCoefficientUnits=N/(m/s)  PyTorqueActuationMode=NoTorque  PyMotionActuationMode=ComputedMotion  PySensePosition=on  PySenseVelocity=off  PySenseAcceleration=off  PySenseTorqueForce=off  PySenseLowerLimitTorqueForce=off  PySenseUpperLimitTorqueForce=off  PyLowerLimitSpecify=off  PyLowerLimitBound=-1  PyLowerLimitBoundUnits=m  PyLowerLimitStiffness=1e6  PyLowerLimitStiffnessUnits=N/m  PyLowerLimitDamping=1e3  PyLowerLimitDampingUnits=N/(m/s)  PyLowerLimitTransitionRegionWidth=1e-4  PyLowerLimitTransitionRegionWidthUnits=m  PyUpperLimitSpecify=off  PyUpperLimitBound=1  PyUpperLimitBoundUnits=m  PyUpperLimitStiffness=1e6  PyUpperLimitStiffnessUnits=N/m  PyUpperLimitDamping=1e3  PyUpperLimitDampingUnits=N/(m/s)  PyUpperLimitTransitionRegionWidth=1e-4  PyUpperLimitTransitionRegionWidthUnits=m  PyPositionTargetSpecify=off  PyPositionTargetPriority=High  PyPositionTargetValue=0  PyPositionTargetValueUnits=m  PyVelocityTargetSpecify=off  PyVelocityTargetPriority=High  PyVelocityTargetValue=0  PyVelocityTargetValueUnits=m/s  PzEquilibriumPosition=0  PzEquilibriumPositionUnits=m  PzSpringStiffness=0  PzSpringStiffnessUnits=N/m  PzDampingCoefficient=0  PzDampingCoefficientUnits=N/(m/s)  PzTorqueActuationMode=NoTorque  PzMotionActuationMode=ComputedMotion  PzSensePosition=on  PzSenseVelocity=off  PzSenseAcceleration=off  PzSenseTorqueForce=off  PzSenseLowerLimitTorqueForce=off  PzSenseUpperLimitTorqueForce=off  PzLowerLimitSpecify=off  PzLowerLimitBound=-1  PzLowerLimitBoundUnits=m  PzLowerLimitStiffness=1e6  PzLowerLimitStiffnessUnits=N/m  PzLowerLimitDamping=1e3  PzLowerLimitDampingUnits=N/(m/s)  PzLowerLimitTransitionRegionWidth=1e-4  PzLowerLimitTransitionRegionWidthUnits=m  PzUpperLimitSpecify=off  PzUpperLimitBound=1  PzUpperLimitBoundUnits=m  PzUpperLimitStiffness=1e6  PzUpperLimitStiffnessUnits=N/m  PzUpperLimitDamping=1e3  PzUpperLimitDampingUnits=N/(m/s)  PzUpperLimitTransitionRegionWidth=1e-4  PzUpperLimitTransitionRegionWidthUnits=m  PzPositionTargetSpecify=off  PzPositionTargetPriority=High  PzPositionTargetValue=0  PzPositionTargetValueUnits=m  PzVelocityTargetSpecify=off  PzVelocityTargetPriority=High  PzVelocityTargetValue=0  PzVelocityTargetValueUnits=m/s  RxEquilibriumPosition=0  RxEquilibriumPositionUnits=deg  RxSpringStiffness=0  RxSpringStiffnessUnits=N*m/deg  RxDampingCoefficient=0  RxDampingCoefficientUnits=N*m/(deg/s)  RxTorqueActuationMode=NoTorque  RxMotionActuationMode=ComputedMotion  RxSensePosition=on  RxSenseVelocity=off  RxSenseAcceleration=off  RxSenseTorqueForce=off  RxSenseLowerLimitTorqueForce=off  RxSenseUpperLimitTorqueForce=off  RxLowerLimitSpecify=off  RxLowerLimitBound=-90  RxLowerLimitBoundUnits=deg  RxLowerLimitStiffness=1e4  RxLowerLimitStiffnessUnits=N*m/deg  RxLowerLimitDamping=10  RxLowerLimitDampingUnits=N*m/(deg/s)  RxLowerLimitTransitionRegionWidth=0.1  RxLowerLimitTransitionRegionWidthUnits=deg  RxUpperLimitSpecify=off  RxUpperLimitBound=90  RxUpperLimitBoundUnits=deg  RxUpperLimitStiffness=1e4  RxUpperLimitStiffnessUnits=N*m/deg  RxUpperLimitDamping=10  RxUpperLimitDampingUnits=N*m/(deg/s)  RxUpperLimitTransitionRegionWidth=0.1  RxUpperLimitTransitionRegionWidthUnits=deg  RxPositionTargetSpecify=off  RxPositionTargetPriority=High  RxPositionTargetValue=0  RxPositionTargetValueUnits=deg  RxVelocityTargetSpecify=off  RxVelocityTargetPriority=High  RxVelocityTargetValue=0  RxVelocityTargetValueUnits=deg/s  RyEquilibriumPosition=0  RyEquilibriumPositionUnits=deg  RySpringStiffness=0  RySpringStiffnessUnits=N*m/deg  RyDampingCoefficient=0  RyDampingCoefficientUnits=N*m/(deg/s)  RyTorqueActuationMode=NoTorque  RyMotionActuationMode=ComputedMotion  RySensePosition=off  RySenseVelocity=off  RySenseAcceleration=off  RySenseTorqueForce=off  RySenseLowerLimitTorqueForce=off  RySenseUpperLimitTorqueForce=off  RyLowerLimitSpecify=off  RyLowerLimitBound=-90  RyLowerLimitBoundUnits=deg  RyLowerLimitStiffness=1e4  RyLowerLimitStiffnessUnits=N*m/deg  RyLowerLimitDamping=10  RyLowerLimitDampingUnits=N*m/(deg/s)  RyLowerLimitTransitionRegionWidth=0.1  RyLowerLimitTransitionRegionWidthUnits=deg  RyUpperLimitSpecify=off  RyUpperLimitBound=90  RyUpperLimitBoundUnits=deg  RyUpperLimitStiffness=1e4  RyUpperLimitStiffnessUnits=N*m/deg  RyUpperLimitDamping=10  RyUpperLimitDampingUnits=N*m/(deg/s)  RyUpperLimitTransitionRegionWidth=0.1  RyUpperLimitTransitionRegionWidthUnits=deg  RyPositionTargetSpecify=off  RyPositionTargetPriority=High  RyPositionTargetValue=0  RyPositionTargetValueUnits=deg  RyVelocityTargetSpecify=off  RyVelocityTargetPriority=High  RyVelocityTargetValue=0  RyVelocityTargetValueUnits=deg/s  RzEquilibriumPosition=0  RzEquilibriumPositionUnits=deg  RzSpringStiffness=0  RzSpringStiffnessUnits=N*m/deg  RzDampingCoefficient=0  RzDampingCoefficientUnits=N*m/(deg/s)  RzTorqueActuationMode=NoTorque  RzMotionActuationMode=ComputedMotion  RzSensePosition=off  RzSenseVelocity=off  RzSenseAcceleration=off  RzSenseTorqueForce=off  RzSenseLowerLimitTorqueForce=off  RzSenseUpperLimitTorqueForce=off  RzLowerLimitSpecify=off  RzLowerLimitBound=-90  RzLowerLimitBoundUnits=deg  RzLowerLimitStiffness=1e4  RzLowerLimitStiffnessUnits=N*m/deg  RzLowerLimitDamping=10  RzLowerLimitDampingUnits=N*m/(deg/s)  RzLowerLimitTransitionRegionWidth=0.1  RzLowerLimitTransitionRegionWidthUnits=deg  RzUpperLimitSpecify=off  RzUpperLimitBound=90  RzUpperLimitBoundUnits=deg  RzUpperLimitStiffness=1e4  RzUpperLimitStiffnessUnits=N*m/deg  RzUpperLimitDamping=10  RzUpperLimitDampingUnits=N*m/(deg/s)  RzUpperLimitTransitionRegionWidth=0.1  RzUpperLimitTransitionRegionWidthUnits=deg  RzPositionTargetSpecify=off  RzPositionTargetPriority=High  RzPositionTargetValue=0  RzPositionTargetValueUnits=deg  RzVelocityTargetSpecify=off  RzVelocityTargetPriority=High  RzVelocityTargetValue=0  RzVelocityTargetValueUnits=deg/s
  TLF Flex : Subsystem  Commented=on
  Transform Sensor{,1..4} (5 alike) : sm_lib/Frames and Transforms/Transform Sensor  MeasurementFrame=World  RotationSequence=XYX  SenseAngle=off  SenseAxis=off  SenseQ=off  SenseR=off  SenseRotationSequence=off  SenseOmegaX=off  SenseOmegaY=off  SenseOmegaZ=off  SenseQDot=off  SenseRDot=off  SenseRotationSequenceDot=off  SenseAlphaX=off  SenseAlphaY=off  SenseAlphaZ=off  SenseQDDot=off  SenseRDDot=off  SenseX=off  SenseY=off  SenseZ=off  SenseRad=off  SenseAzim=off  SenseDist=on  SenseInc=off  SenseXDot=off  SenseYDot=off  SenseZDot=off  SenseRadDot=off  SenseAzimDot=off  SenseDistDot=off  SenseIncDot=off  SenseXDDot=off  SenseYDDot=off  SenseZDDot=off  SenseRadDDot=off  SenseAzimDDot=off  SenseDistDDot=off  SenseIncDDot=off
  Weld Joint{,1..9} (10 alike) : sm_lib/Joints/Weld Joint  JointMode=Normal  SenseConstraintForce=off  SenseConstraintForceX=off  SenseConstraintForceY=off  SenseConstraintForceZ=off  SenseConstraintTorque=off  SenseConstraintTorqueX=off  SenseConstraintTorqueY=off  SenseConstraintTorqueZ=off  SenseTotalForce=on  SenseTotalForceX=off  SenseTotalForceY=off  SenseTotalForceZ=off  SenseTotalTorque=on  SenseTotalTorqueX=off  SenseTotalTorqueY=off  SenseTotalTorqueZ=off  CompositeWrenchDir=FollowerOnBase  CompositeWrenchFrame=BaseFrame
  World Frame : sm_lib/Frames and Transforms/World Frame
  Left Psoas force : Outport  OutDataTypeStr=double  PortDimensions=[1 1]  SampleTime=0
  Left MF force : Outport  Port=2  OutDataTypeStr=double  PortDimensions=[1 1]  SampleTime=0
  Left LongThor force : Outport  Port=3  OutDataTypeStr=double  PortDimensions=[1 1]  SampleTime=0
  Left EO force : Outport  Port=4  OutDataTypeStr=double  PortDimensions=[1 1]  SampleTime=0
  Left IO force : Outport  Port=5  OutDataTypeStr=double  PortDimensions=[1 1]  SampleTime=0
  Left RA force : Outport  Port=6  OutDataTypeStr=double  PortDimensions=[1 1]  SampleTime=0
  Force on L1 by AbdFlex : Outport  Port=7  OutDataTypeStr=double  PortDimensions=1
  Force on L2 by AbdFlex : Outport  Port=8  OutDataTypeStr=double  PortDimensions=1
  Force on L3 by AbdFlex : Outport  Port=9  OutDataTypeStr=double  PortDimensions=1
  Force on L4 by AbdFlex : Outport  Port=10  OutDataTypeStr=double  PortDimensions=1
  Force on L5 by AbdFlex : Outport  Port=11  OutDataTypeStr=double  PortDimensions=1
  output : Outport  Port=12  OutDataTypeStr=double  PortDimensions=[3 1]  SampleTime=0
  output1 : Outport  Port=13  OutDataTypeStr=double  PortDimensions=[1 1]  SampleTime=0
  output2 : Outport  Port=14  OutDataTypeStr=double  PortDimensions=[3 1]  SampleTime=0
  output3 : Outport  Port=15  OutDataTypeStr=double  PortDimensions=[1 1]  SampleTime=0
  output4 : Outport  Port=16  OutDataTypeStr=double  PortDimensions=[3 1]  SampleTime=0
  output5 : Outport  Port=17  OutDataTypeStr=double  PortDimensions=[1 1]  SampleTime=0
  output6 : Outport  Port=18  OutDataTypeStr=double  PortDimensions=[1 1]  SampleTime=0
  output7 : Outport  Port=19  OutDataTypeStr=double  PortDimensions=[3 1]  SampleTime=0
  output8 : Outport  Port=20  OutDataTypeStr=double  PortDimensions=[1 1]  SampleTime=0
  output9 : Outport  Port=21  OutDataTypeStr=double  PortDimensions=[1 1]  SampleTime=0
  output10 : Outport  Port=22  OutDataTypeStr=double  PortDimensions=[3 1]  SampleTime=0
  output11 : Outport  Port=23  OutDataTypeStr=double  PortDimensions=[1 1]  SampleTime=0
  output12 : Outport  Port=24  OutDataTypeStr=double  PortDimensions=[3 1]  SampleTime=0
  output13 : Outport  Port=25  OutDataTypeStr=double  PortDimensions=[3 1]  SampleTime=0
  output14 : Outport  Port=26  OutDataTypeStr=double  PortDimensions=[3 1]  SampleTime=0
  output15 : Outport  Port=27  OutDataTypeStr=double  PortDimensions=[1 1]  SampleTime=0
  output16 : Outport  Port=28  OutDataTypeStr=double  PortDimensions=[3 1]  SampleTime=0
  output17 : Outport  Port=29  OutDataTypeStr=double  PortDimensions=[3 1]  SampleTime=0
  output18 : Outport  Port=30  OutDataTypeStr=double  PortDimensions=[3 1]  SampleTime=0
  output19 : Outport  Port=31  OutDataTypeStr=double  PortDimensions=[3 1]  SampleTime=0
  output20 : Outport  Port=32  OutDataTypeStr=double  PortDimensions=[3 1]  SampleTime=0
  output21 : Outport  Port=33  OutDataTypeStr=double  PortDimensions=[3 1]  SampleTime=0
  output22 : Outport  Port=34  OutDataTypeStr=double  PortDimensions=[3 1]  SampleTime=0
  output23 : Outport  Port=35  OutDataTypeStr=double  PortDimensions=[3 1]  SampleTime=0
  output24 : Outport  Port=36  OutDataTypeStr=double  PortDimensions=[3 1]  SampleTime=0
  output25 : Outport  Port=37  OutDataTypeStr=double  PortDimensions=[3 1]  SampleTime=0
  output26 : Outport  Port=38  OutDataTypeStr=double  PortDimensions=[3 1]  SampleTime=0
  output27 : Outport  Port=39  OutDataTypeStr=double  PortDimensions=[3 1]  SampleTime=0
  px : Outport  Port=40  OutDataTypeStr=double  PortDimensions=[1 1]  SampleTime=0
  py : Outport  Port=41  OutDataTypeStr=double  PortDimensions=[1 1]  SampleTime=0
  pz : Outport  Port=42  OutDataTypeStr=double  PortDimensions=[1 1]  SampleTime=0
  qx : Outport  Port=43  OutDataTypeStr=double  PortDimensions=[1 1]  SampleTime=0
  wires:
  PS-Simulink Converter27/1 -> output4/1
  input0/1 -> Simulink-PS Converter7/1  "Downward force at T1"
  input2/1 -> Simulink-PS Converter1/1  "Flexion force at L1"
  Constant13/1 -> Subtract2/2
  IAP - AbdFlex/1(Outport) -> Force on L1 by AbdFlex/1  "Force on L1 by AbdFlex"
  PS-Simulink Converter28/1 -> output7/1
  PS-Simulink Converter9/1 -> output5/1
  PS-Simulink Converter33/1 -> output22/1
  PS-Simulink Converter31/1 -> output16/1
  input5/1 -> Simulink-PS Converter2/1  "Pure FE Moment at L1 COM"
  PS-Simulink Converter21/1 -> output14/1
  PS-Simulink Converter10/1 -> output3/1
  PS-Simulink Converter24/1 -> Gain16/1
  PS-Simulink Converter25/1 -> Gain17/1
  Radians to Degrees3/1 -> Add5/1, Scope5/1
  PS-Simulink Converter35/1 -> Radians to Degrees9/1
  "Left RA "/1 -> Muscle Forces/12("Left RA ")
  Subtract2/1 -> L3-L4 disc height1/1, Scope17/3
  Constant5/1 -> Simulink-PS Converter/1
  "Left LongThor "/1 -> Muscle Forces/6("Left LongThor ")
  Gain18/1 -> Subtract4/1
  PS-Simulink Converter22/1 -> Gain14/1
  PS-Simulink Converter1/1 -> output6/1
  input3/1 -> Simulink-PS Converter3/1  "Pure LB Moment at L1 COM"
  PS-Simulink Converter14/1 -> output23/1
  Subtract/1 -> L5-S1 disc height/1, Scope17/5
  Subtract1/1 -> L4-L5 disc height1/1, Scope17/4
  Gain16/1 -> Subtract2/1
  "Right MF "/1 -> Muscle Forces/3("Right MF ")
  Subtract4/1 -> Scope17/1, L1-L2 disc height1/1
  "Right Psoas "/1 -> Muscle Forces/1("Right Psoas ")
  Gain15/1 -> Subtract1/1
  Constant11/1 -> Subtract/2
  PS-Simulink Converter11/1 -> output8/1
  PS-Simulink Converter23/1 -> Gain15/1
  "Right LongThor "/1 -> Muscle Forces/5("Right LongThor ")
  Subtract3/1 -> L2-L3 disc height2/1, Scope17/2
  Gain14/1 -> Subtract/1
  PS-Simulink Converter13/1 -> output15/1
  Constant15/1 -> Subtract4/2
  Add5/1 -> Gain4/1
  Radians to Degrees9/1 -> Add20/1, Scope19/1
  PS-Simulink Converter8/1 -> Radians to Degrees3/1
  Gain17/1 -> Subtract3/1
  PS-Simulink Converter18/1 -> output17/1
  Muscle Forces/4(Left EO force) -> Left EO force/1  "Left EO"
  Add20/1 -> Gain19/1
  Gain19/1 -> Scope20/1, L1-S1 Moment-Rotation/2  "L1-S1 rot"
  Muscle Forces/3(Left LongThor force) -> Left LongThor force/1  "Left LongThor"
  PS-Simulink Converter4/1 -> output2/1
  PS-Simulink Converter20/1 -> output13/1
  IAP - AbdFlex/3(Outport2) -> Force on L3 by AbdFlex/1  "Force on L3 by AbdFlex"
  Constant12/1 -> Subtract1/2
  Constant1/1 -> Add5/2
  PS-Simulink Converter34/1 -> output25/1
  IAP - AbdFlex/2(Outport1) -> Force on L2 by AbdFlex/1  "Force on L2 by AbdFlex"
  PS-Simulink Converter39/1 -> qx/1  "qx"
  Muscle Forces/1(Left Psoas force) -> Left Psoas force/1  "Left Psoas"
  "Right EO "/1 -> Muscle Forces/7("Right EO ")
  PS-Simulink Converter2/1 -> output26/1
  IAP - AbdFlex/4(Outport3) -> Force on L4 by AbdFlex/1  "Force on L4 by AbdFlex"
  PS-Simulink Converter/1 -> output1/1
  PS-Simulink Converter29/1 -> output10/1
  PS-Simulink Converter15/1 -> output24/1
  "Left IO "/1 -> Muscle Forces/10("Left IO ")
  Gain4/1 -> Scope6/1  "L5-S1 FE Rot"
  Multiply21/1 -> Simulink-PS Converter5/1
  PS-Simulink Converter32/1 -> output19/1
  PS-Simulink Converter36/1 -> px/1  "px"
  Gain20/1 -> L1-S1 Moment-Rotation/1  "L1-S1 moment"
  "Left MF "/1 -> Muscle Forces/4("Left MF ")
  In22/1 -> Gain20/1  "Pure FE Moment at L1 COM"
  "Right IO "/1 -> Muscle Forces/9("Right IO ")
  In13/1 -> TLF Flex/1(In1)
  PS-Simulink Converter26/1 -> Gain18/1
  Constant14/1 -> Subtract3/2
  PS-Simulink Converter3/1 -> output/1
  input1/1 -> Simulink-PS Converter6/1  "Forward force at T1"
  Constant16/1 -> Add20/2
  PS-Simulink Converter16/1 -> output20/1
  PS-Simulink Converter5/1 -> output9/1
  PS-Simulink Converter6/1 -> output27/1
  Muscle Forces/5(Left IO force) -> Left IO force/1  "Left IO"
  Muscle Forces/6(Left RA force) -> Left RA force/1  "Left RA"
  input4/1 -> Simulink-PS Converter4/1  "Pure AR Moment at L1 COM"
  Muscle Forces/2(Left MF force) -> Left MF force/1  "Left MF"
  PS-Simulink Converter17/1 -> output21/1
  IAP - AbdFlex/5(Outport4) -> Force on L5 by AbdFlex/1  "Force on L5 by AbdFlex"
  PS-Simulink Converter12/1 -> output11/1
  PS-Simulink Converter30/1 -> output12/1
  PS-Simulink Converter19/1 -> output18/1
  PS-Simulink Converter37/1 -> py/1  "py"
  PS-Simulink Converter38/1 -> pz/1  "pz"
  Left Psoas/1 -> Muscle Forces/2(Left Psoas)
  "Left EO "/1 -> Muscle Forces/8("Left EO ")
  In14/1 -> TLF Flex/2(In2)
  In15/1 -> Multiply21/1
  "Right RA "/1 -> Muscle Forces/11("Right RA ")
  connections:
  L1-S1 movement/LConn1 -- Weld Joint/LConn1 -- S1/LConn1 -- L5-S1 follower load/LConn1 -- L5-S1 follower load1/RConn1 -- Transform Sensor/LConn1 -- L5-S1 movement/LConn1
  Muscle Forces/LConn2 -- S1/RConn2 -- Muscle Forces/LConn67
  Weld Joint2/LConn1 -- L4/RConn1 -- L3-L4 movement/LConn1 -- Transform Sensor2/LConn1 -- L3-L4 follower load2/LConn1
  Simulink-PS Converter5/RConn1 -- L1-L2 follower load1/LConn2 -- L2-L3 follower load1/LConn2 -- L3-L4 follower load1/LConn2 -- L4-L5 follower load1/LConn2 -- L5-S1 follower load1/LConn2
  L5/RConn6 -- Muscle Forces/LConn33 -- TLF Flex/LConn4
  Muscle Forces/LConn27 -- L3/RConn6 -- TLF Flex/LConn2
  L3/RConn1 -- Weld Joint3/LConn1 -- L2-L3 movement/LConn1 -- L2-L3 follower load3/LConn1 -- Transform Sensor3/LConn1
  Simulink-PS Converter/RConn1 -- L5-S1 follower load/LConn2 -- L4-L5 follower load/LConn2 -- L3-L4 follower load2/LConn2 -- L2-L3 follower load3/LConn2 -- L1-L2 follower load4/LConn2
  Muscle Forces/LConn9 -- World Frame/RConn1 -- Mechanism Configuration/RConn1 -- Solver Configuration/RConn1 -- S1/RConn1 -- Supraspinous Ligaments/RConn1 -- Interspinous Ligaments/LConn11 -- TLF Flex/LConn8
  Muscle Forces/LConn20 -- L1/RConn4 -- TLF Flex/LConn3
  L2-L3 follower load1/RConn1 -- AdbFlex_L3 mount/LConn2 -- L3-L4 follower load1/LConn1
  AbdFlex_L4 mount/LConn1 -- IAP - AbdFlex/LConn3 -- L4/LConn1 -- Weld Joint9/RConn1 -- L4-L5 movement/RConn1 -- Transform Sensor1/RConn1 -- L4-L5 follower load/RConn1
  L2/LConn1 -- Weld Joint7/RConn1 -- L2-L3 movement/RConn1 -- Transform Sensor3/RConn1 -- L2-L3 follower load3/RConn1 -- AbdFlex_L2 mount/LConn1 -- IAP - AbdFlex/LConn5
  Weld Joint4/LConn1 -- L2/RConn1 -- Bushing Joint2/LConn1 -- L1-L2 follower load4/LConn1 -- Transform Sensor4/LConn1 -- L1-L2 movement/LConn1
  Muscle Forces/LConn25 -- L2/RConn6 -- TLF Flex/LConn5
  L1-L2 follower load1/RConn1 -- AbdFlex_L2 mount/LConn2 -- L2-L3 follower load1/LConn1
  L5/LConn1 -- Weld Joint5/RConn1 -- AbdFlex_L5 mount/LConn1 -- IAP - AbdFlex/LConn2 -- Transform Sensor/RConn1 -- L5-S1 follower load/RConn1
  Flexion force at L1/RConn1 -- Pure LB Moment at L1 COM/RConn1 -- Pure AR Moment at L1 COM/RConn1 -- Pure FE Moment at L1 COM/RConn1 -- L1/RConn1 -- IAP - Individual Forces Model/LConn1 -- IAP - AbdFlex/LConn7 -- L1-S1 movement/RConn1 -- Left T Spine/LConn1 -- Right T Spine/LConn1 -- Bushing Joint/RConn1
  L3/LConn1 -- Weld Joint8/RConn1 -- Transform Sensor2/RConn1 -- L3-L4 follower load2/RConn1 -- L3-L4 movement/RConn1 -- AdbFlex_L3 mount/LConn1 -- IAP - AbdFlex/LConn4
  L5-S1 movement/RConn1 -- L5/LConn2 -- IAP - Individual Forces Model/RConn1
  L5/RConn1 -- Weld Joint1/LConn1 -- L4-L5 movement/LConn1 -- Transform Sensor1/LConn1 -- L4-L5 follower load/LConn1
  Muscle Forces/LConn30 -- L4/RConn6 -- TLF Flex/LConn1
  L4-L5 follower load1/RConn1 -- AbdFlex_L5 mount/LConn2 -- L5-S1 follower load1/LConn1
  L3-L4 follower load1/RConn1 -- AbdFlex_L4 mount/LConn2 -- L4-L5 follower load1/LConn1
  Muscle Forces/LConn1 -- S1/LConn6 -- Muscle Forces/LConn68
  Muscle Forces/RConn1 -- Right T Spine/RConn1 -- Muscle Forces/LConn65
  Forward force at T1/RConn1 -- Right T Spine/RConn3 -- T1-S1 Bushing Joint/RConn1 -- Downward force at T1/RConn1
  Bushing Joint/LConn1 -- S1/LConn2 -- IAP - AbdFlex/LConn1 -- T1-S1 Bushing Joint/LConn1
  L1/LConn1 -- Weld Joint6/RConn1 -- Bushing Joint2/RConn1 -- Transform Sensor4/RConn1 -- L1-L2 follower load4/RConn1 -- L1-L2 movement/RConn1 -- AdbFlex_L1 mount/LConn1 -- IAP - AbdFlex/LConn6
  Muscle Forces/RConn5 -- Left T Spine/RConn1 -- Muscle Forces/LConn66
  Hand with cube/RConn1 -- TLF Flex/RConn5 -- Right T Spine/RConn8
  Left and Right Intertransverse Ligaments/LConn14 -- L3/RConn5
  L4/LConn9 -- Muscle Forces/LConn29
  TLF Flex/RConn7 -- Right T Spine/LConn10
  Left and Right Intertransverse Ligaments/LConn7 -- L4/LConn5
  TLF Flex/RConn2 -- Left T Spine/RConn6
  Weld Joint3/RConn3 -- PS-Simulink Converter31/LConn1
  TLF Flex/RConn3 -- Left T Spine/LConn7
  IVD2/RConn1 -- Weld Joint7/LConn1
  L3/RConn7 -- Muscle Forces/LConn17
  IVD5/LConn1 -- Weld Joint/RConn1
  TLF Flex/LConn6 -- Left T Spine/RConn7
  L1/RConn7 -- Muscle Forces/LConn22
  TLF Flex/LConn7 -- Left T Spine/RConn8
  Pure LB Moment at L1 COM/LConn1 -- Simulink-PS Converter3/RConn1
  Weld Joint1/RConn3 -- PS-Simulink Converter27/LConn1
  L1/LConn6 -- Muscle Forces/LConn35
  Interspinous Ligaments/LConn9 -- L2/LConn4
  Left T Spine/LConn6 -- TLF Flex/RConn1
  Left and Right Intertransverse Ligaments/LConn12 -- L3/LConn6
  Weld Joint4/RConn3 -- PS-Simulink Converter33/LConn1
  Left and Right Intertransverse Ligaments/LConn18 -- L2/RConn5
  Muscle Forces/LConn47 -- Right T Spine/RConn6
  Weld Joint6/RConn2 -- PS-Simulink Converter21/LConn1
  Muscle Forces/LConn54 -- Right T Spine/RConn7
  Muscle Forces/LConn23 -- L2/LConn9
  PS-Simulink Converter6/LConn1 -- Weld Joint5/RConn2
  TLF Flex/LConn9 -- Right T Spine/RConn9
  L4/RConn9 -- Muscle Forces/LConn31
  Supraspinous Ligaments/LConn2 -- S1/RConn6
  L5/LConn7 -- Muscle Forces/LConn15
  TLF Flex/LConn10 -- Right T Spine/RConn10
  L2/RConn8 -- Muscle Forces/LConn41
  TLF Flex/RConn4 -- Left T Spine/LConn8
  TLF Flex/RConn8 -- Right T Spine/LConn11
  L2/RConn7 -- Muscle Forces/LConn16
  TLF Flex/RConn6 -- Right T Spine/LConn9
  Supraspinous Ligaments/LConn7 -- L3/RConn3
  Weld Joint4/RConn2 -- PS-Simulink Converter20/LConn1
  Interspinous Ligaments/LConn3 -- L5/LConn4
  L1-L2 movement/RConn5 -- PS-Simulink Converter13/LConn1
  L1-L2 follower load1/LConn1 -- AdbFlex_L1 mount/LConn2
  Interspinous Ligaments/LConn2 -- L5/RConn2
  PS-Simulink Converter38/LConn1 -- T1-S1 Bushing Joint/RConn4
  L4/RConn7 -- Muscle Forces/LConn18
  Left and Right Intertransverse Ligaments/LConn1 -- S1/RConn7
  Left and Right Intertransverse Ligaments/LConn4 -- L5/LConn5
  Muscle Forces/LConn51 -- S1/RConn8
  Muscle Forces/LConn49 -- S1/RConn9
  Muscle Forces/LConn28 -- L3/RConn9
  IAP - Individual Forces Model/RConn4 -- L3/LConn2
  Left and Right Intertransverse Ligaments/LConn6 -- L5/RConn5
  Muscle Forces/LConn19 -- L5/RConn7
  Muscle Forces/LConn53 -- Right T Spine/LConn7
  S1/LConn13 -- Muscle Forces/LConn64
  L3/RConn8 -- Muscle Forces/LConn42
  Muscle Forces/RConn6 -- Left T Spine/LConn2
  Weld Joint3/RConn2 -- PS-Simulink Converter18/LConn1
  Left and Right Intertransverse Ligaments/LConn11 -- L3/LConn5
  S1/LConn12 -- Muscle Forces/LConn62
  Weld Joint1/RConn1 -- IVD4/LConn1
  Weld Joint2/RConn2 -- PS-Simulink Converter16/LConn1
  Bushing Joint/RConn2 -- PS-Simulink Converter9/LConn1
  Left T Spine/RConn4 -- Muscle Forces/LConn56
  Weld Joint2/RConn3 -- PS-Simulink Converter29/LConn1
  PS-Simulink Converter22/LConn1 -- Transform Sensor/RConn2
  L2/LConn8 -- Muscle Forces/LConn37
  IAP - Individual Forces Model/RConn3 -- L2/LConn2
  PS-Simulink Converter23/LConn1 -- Transform Sensor1/RConn2
  L4/RConn8 -- Muscle Forces/LConn43
  Muscle Forces/LConn45 -- Right T Spine/LConn6
  Muscle Forces/LConn4 -- S1/LConn4
  PS-Simulink Converter24/LConn1 -- Transform Sensor2/RConn2
  Muscle Forces/LConn50 -- S1/LConn10
  Supraspinous Ligaments/LConn5 -- L4/RConn3
  Muscle Forces/LConn48 -- Left T Spine/LConn4
  Bushing Joint/RConn4 -- PS-Simulink Converter5/LConn1
  PS-Simulink Converter26/LConn1 -- Transform Sensor4/RConn2
  Muscle Forces/LConn5 -- S1/LConn3
  Interspinous Ligaments/LConn10 -- L1/RConn2
  PS-Simulink Converter2/LConn1 -- Weld Joint/RConn2
  Supraspinous Ligaments/LConn8 -- L2/LConn3
  PS-Simulink Converter25/LConn1 -- Transform Sensor3/RConn2
  Left and Right Intertransverse Ligaments/LConn16 -- L2/LConn6
  Weld Joint4/RConn1 -- IVD1/LConn1
  Muscle Forces/LConn7 -- S1/RConn5
  IVD4/RConn1 -- Weld Joint9/LConn1
  L5-S1 movement/RConn5 -- PS-Simulink Converter/LConn1
  Left and Right Intertransverse Ligaments/LConn19 -- L1/LConn4
  Weld Joint9/RConn3 -- PS-Simulink Converter28/LConn1
  Weld Joint7/RConn2 -- PS-Simulink Converter19/LConn1
  Simulink-PS Converter4/RConn1 -- Pure AR Moment at L1 COM/LConn1
  Weld Joint8/RConn3 -- PS-Simulink Converter30/LConn1
  Weld Joint6/RConn3 -- PS-Simulink Converter34/LConn1
  Left and Right Intertransverse Ligaments/LConn10 -- L4/RConn5
  Weld Joint7/RConn3 -- PS-Simulink Converter32/LConn1
  L5/RConn9 -- Muscle Forces/LConn34
  L2/LConn7 -- Muscle Forces/LConn12
  Muscle Forces/LConn59 -- S1/RConn10
  T1-S1 Bushing Joint/RConn5 -- PS-Simulink Converter39/LConn1
  PS-Simulink Converter8/LConn1 -- Bushing Joint2/RConn5
  Muscle Forces/LConn46 -- Left T Spine/RConn3
  L4/LConn8 -- Muscle Forces/LConn39
  Flexion force at L1/LConn1 -- Simulink-PS Converter1/RConn1
  Bushing Joint/RConn3 -- PS-Simulink Converter1/LConn1
  Interspinous Ligaments/LConn7 -- L2/RConn2
  Supraspinous Ligaments/LConn3 -- L5/RConn3
  IAP - Individual Forces Model/RConn2 -- L4/LConn2
  Left and Right Intertransverse Ligaments/LConn3 -- L5/LConn6
  IAP - Individual Forces Model/RConn5 -- L1/LConn2
  Interspinous Ligaments/LConn8 -- L3/LConn4
  Muscle Forces/LConn3 -- S1/RConn4
  Weld Joint3/RConn1 -- IVD2/LConn1
  Weld Joint2/RConn1 -- IVD3/LConn1
  Left and Right Intertransverse Ligaments/LConn9 -- L4/RConn4
  Left and Right Intertransverse Ligaments/LConn8 -- L4/LConn6
  Left and Right Intertransverse Ligaments/LConn5 -- L5/RConn4
  Left and Right Intertransverse Ligaments/LConn2 -- S1/LConn8
  L3/LConn7 -- Muscle Forces/LConn13
  Left and Right Intertransverse Ligaments/LConn13 -- L3/RConn4
  L3/LConn8 -- Muscle Forces/LConn38
  PS-Simulink Converter4/LConn1 -- Weld Joint5/RConn3
  PS-Simulink Converter11/LConn1 -- L3-L4 movement/RConn5
  Supraspinous Ligaments/LConn10 -- L1/LConn3
  Simulink-PS Converter2/RConn1 -- Pure FE Moment at L1 COM/LConn1
  Muscle Forces/RConn4 -- Right T Spine/RConn2
  Supraspinous Ligaments/LConn1 -- L5/LConn3
  Muscle Forces/RConn2 -- Right T Spine/LConn2
  PS-Simulink Converter3/LConn1 -- Weld Joint/RConn3
  Weld Joint5/LConn1 -- IVD5/RConn1
  Muscle Forces/RConn3 -- Right T Spine/LConn3
  L2/RConn9 -- Muscle Forces/LConn24
  IVD1/RConn1 -- Weld Joint6/LConn1
  PS-Simulink Converter10/LConn1 -- L4-L5 movement/RConn5
  Interspinous Ligaments/LConn6 -- L4/LConn4
  Muscle Forces/LConn8 -- S1/LConn5
  IVD3/RConn1 -- Weld Joint8/LConn1
  Left and Right Intertransverse Ligaments/LConn20 -- L1/RConn3
  L2-L3 movement/RConn5 -- PS-Simulink Converter12/LConn1
  Supraspinous Ligaments/LConn4 -- L4/LConn3
  Interspinous Ligaments/LConn4 -- L4/RConn2
  Supraspinous Ligaments/LConn6 -- L3/LConn3
  PS-Simulink Converter14/LConn1 -- Weld Joint1/RConn2
  Forward force at T1/LConn1 -- Simulink-PS Converter6/RConn1
  PS-Simulink Converter37/LConn1 -- T1-S1 Bushing Joint/RConn3
  Interspinous Ligaments/LConn1 -- S1/LConn7
  Muscle Forces/RConn7 -- Left T Spine/RConn2
  L1/RConn6 -- Muscle Forces/LConn36
  PS-Simulink Converter35/LConn1 -- L1-S1 movement/RConn5
  Muscle Forces/LConn21 -- L1/LConn7
  Downward force at T1/LConn1 -- Simulink-PS Converter7/RConn1
  Left T Spine/RConn5 -- Muscle Forces/LConn58
  L5/LConn8 -- Muscle Forces/LConn40
  Muscle Forces/LConn61 -- S1/RConn11
  Left and Right Intertransverse Ligaments/LConn17 -- L2/RConn4
  Left and Right Intertransverse Ligaments/LConn15 -- L2/LConn5
  Supraspinous Ligaments/LConn9 -- L2/RConn3
  Muscle Forces/LConn55 -- Right T Spine/LConn8
  L4/LConn7 -- Muscle Forces/LConn14
  L1/LConn5 -- Muscle Forces/LConn10
  L1/RConn5 -- Muscle Forces/LConn11
  Muscle Forces/LConn26 -- L3/LConn9
  Muscle Forces/LConn57 -- Left T Spine/LConn5
  S1/LConn9 -- Muscle Forces/LConn52
  Weld Joint8/RConn2 -- PS-Simulink Converter17/LConn1
  S1/LConn11 -- Muscle Forces/LConn60
  Muscle Forces/RConn8 -- Left T Spine/LConn3
  Muscle Forces/LConn63 -- S1/RConn12
  L5/LConn9 -- Muscle Forces/LConn32
  Muscle Forces/LConn6 -- S1/RConn3
  L5/RConn8 -- Muscle Forces/LConn44
  PS-Simulink Converter15/LConn1 -- Weld Joint9/RConn2
  PS-Simulink Converter36/LConn1 -- T1-S1 Bushing Joint/RConn2
  Interspinous Ligaments/LConn5 -- L3/RConn2
